simulink model "CarControl"  (R2022b)
settings: Solver=FixedStepDiscrete  StartTime=0.0  StopTime=10.0  FixedStep=0.01  RelTol=1e-3
libraries: simulink x9, simulink_extras x1
settings Model: Creator=Admin  LastModifiedBy=lu
settings OptimizationCC: DefaultParameterBehavior=Inlined  UseDivisionForNetSlopeComputation=on  GainParamInheritBuiltInType=on  UseFloatMulNetSlope=on  InlineInvariantSignals=on  PassReuseOutputArgsAs=Individual arguments  ZeroExternalMemoryAtStartup=off  ZeroInternalMemoryAtStartup=off  NoFixptDivByZeroProtection=on  EfficientFloat2IntCast=on  LifeSpan=1  OptimizeBlockOrder=speed  DifferentSizesBufferReuse=on  EfficientTunableParamExpr=on
settings DebuggingCC: ParameterTunabilityLossMsg=error  UnconnectedInputMsg=warning  UnconnectedOutputMsg=warning  UnconnectedLineMsg=warning
settings HardwareCC: ProdLongLongMode=on
settings SFSimCC: MATLABDynamicMemAlloc=off
settings RTWCC: Description=Embedded Coder  SystemTargetFile=ert.tlc  PackageName=RemoteControllerCodeGen  TemplateMakefile=ert_default_tmf  DLArmComputeVersion=19.05
settings CodeAppCC: ForceParamTrailComments=on  IgnoreCustomStorageClasses=off  OperatorAnnotations=on  SimulinkDataObjDesc=on  SFDataObjDesc=on  CustomSymbolStrGlobalVar=rt$N$M  CustomSymbolStrType=$N$M  CustomSymbolStrFcn=$N$M$F  CustomSymbolStrMacro=$N$M  InsertBlockDesc=on
settings ERTTargetCC: TargetLangStandard=C99 (ISO)  GenerateSampleERTMain=on  IncludeMdlTerminateFcn=off  CombineSignalStateStructs=on  SupportAbsoluteTime=off  SupportComplex=off  SupportNonInlinedSFcns=on  InlinedParameterPlacement=NonHierarchical  ERTCustomFileTemplate=example_file_process.tlc  ERTFilePackagingFormat=CompactWithDataFile

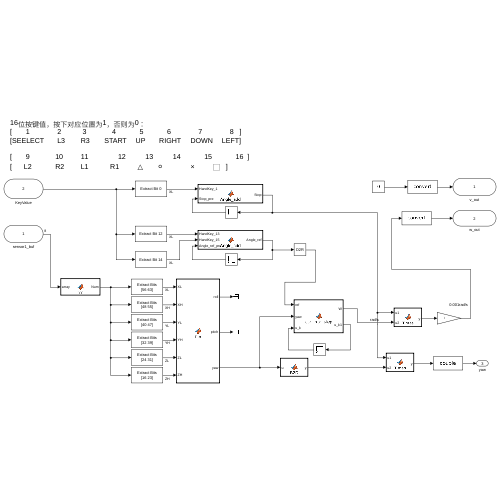
[thumbnail: Simulink's stored preview of the top-level diagram]
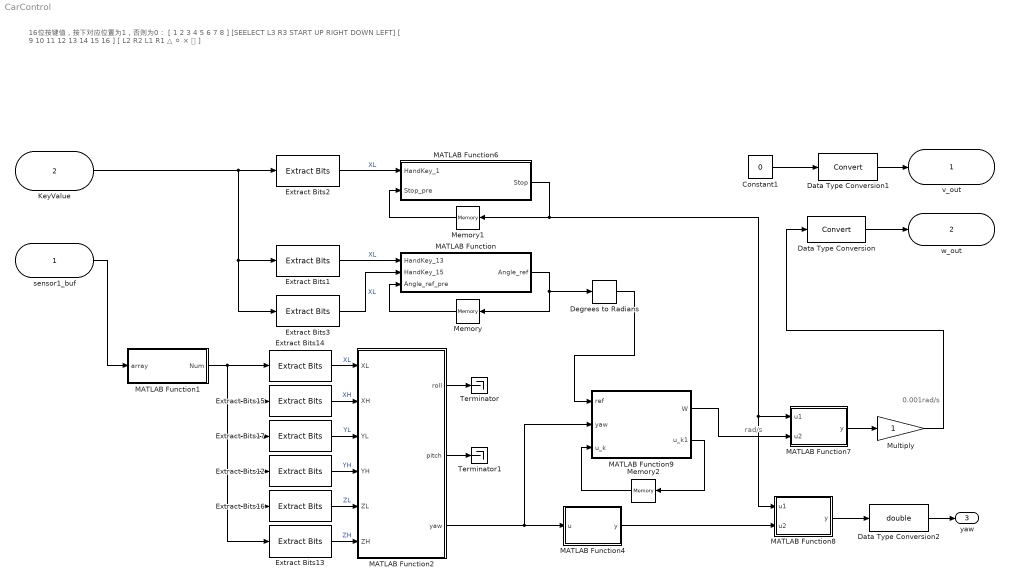
== system CarControl ==
  note: 16位按键值，按下对应位置为1，否则为0：
      | [ 1 2 3 4 5 6 7 8 ]
      | [SEELECT L3 R3 START UP RIGHT DOWN LEFT]
      |
      | [ 9 10 11 12 13 14 15 16 ]
      | [ L2 R2 L1 R1 △ ⚪ × ⃞ ]
  note: 0.001rad/s
  note: rad/s
  sensor1_buf : Inport  OutDataTypeStr=int8  PortDimensions=8
  KeyValue : Inport  Port=2  OutDataTypeStr=uint16  PortDimensions=1
  Constant1 : Constant  Value=0  OutDataTypeStr=uint8  SampleTime=-1
  Data Type Conversion : DataTypeConversion  SaturateOnIntegerOverflow=off  RndMeth=Floor
  Data Type Conversion1 : DataTypeConversion  SaturateOnIntegerOverflow=off  RndMeth=Floor
  Data Type Conversion2 : DataTypeConversion  OutDataTypeStr=double  SaturateOnIntegerOverflow=off  RndMeth=Floor
  Degrees to Radians : simulink_extras/Transformations/Degrees to Radians
  Extract Bits1 : simulink/Logic and Bit Operations/Extract Bits  bitsToExtract=Range of bits  numBits=8  bitIdxRange=[12]  outScalingMode=Treat bit field as an integer
  Extract Bits12 : simulink/Logic and Bit Operations/Extract Bits  bitsToExtract=Range of bits  numBits=8  bitIdxRange=[32 39]  outScalingMode=Treat bit field as an integer
  Extract Bits13 : simulink/Logic and Bit Operations/Extract Bits  bitsToExtract=Range of bits  numBits=8  bitIdxRange=[16 23]  outScalingMode=Treat bit field as an integer
  Extract Bits14 : simulink/Logic and Bit Operations/Extract Bits  bitsToExtract=Range of bits  numBits=8  bitIdxRange=[56 63]  outScalingMode=Treat bit field as an integer
  Extract Bits15 : simulink/Logic and Bit Operations/Extract Bits  bitsToExtract=Range of bits  numBits=8  bitIdxRange=[48 55]  outScalingMode=Treat bit field as an integer
  Extract Bits16 : simulink/Logic and Bit Operations/Extract Bits  bitsToExtract=Range of bits  numBits=8  bitIdxRange=[24 31]  outScalingMode=Treat bit field as an integer
  Extract Bits17 : simulink/Logic and Bit Operations/Extract Bits  bitsToExtract=Range of bits  numBits=8  bitIdxRange=[40 47]  outScalingMode=Treat bit field as an integer
  Extract Bits2 : simulink/Logic and Bit Operations/Extract Bits  bitsToExtract=Range of bits  numBits=8  bitIdxRange=[0]  outScalingMode=Treat bit field as an integer
  Extract Bits3 : simulink/Logic and Bit Operations/Extract Bits  bitsToExtract=Range of bits  numBits=8  bitIdxRange=[14]  outScalingMode=Treat bit field as an integer
  MATLAB Function : MATLAB Function  TreatAsAtomicUnit=on
  MATLAB Function1 : MATLAB Function  TreatAsAtomicUnit=on
  MATLAB Function2 : MATLAB Function  TreatAsAtomicUnit=on
  MATLAB Function4 : MATLAB Function  TreatAsAtomicUnit=on
  MATLAB Function6 : MATLAB Function  TreatAsAtomicUnit=on
  MATLAB Function7 : MATLAB Function  TreatAsAtomicUnit=on
  MATLAB Function8 : MATLAB Function  TreatAsAtomicUnit=on
  MATLAB Function9 : MATLAB Function  TreatAsAtomicUnit=on
  Memory : Memory
  Memory1 : Memory
  Memory2 : Memory
  Multiply : Gain  OutDataTypeStr=double
  Terminator : Terminator
  Terminator1 : Terminator
  v_out : Outport  OutDataTypeStr=double
  w_out : Outport  Port=2  OutDataTypeStr=double
  yaw : Outport  Port=3  OutDataTypeStr=double
  wires:
  Extract Bits14/1 -> MATLAB Function2/1(XL)  "XL"
  Extract Bits15/1 -> MATLAB Function2/2(XH)  "XH"
  Extract Bits17/1 -> MATLAB Function2/3(YL)  "YL"
  Extract Bits13/1 -> MATLAB Function2/6(ZH)  "ZH"
  Extract Bits12/1 -> MATLAB Function2/4(YH)  "YH"
  Extract Bits16/1 -> MATLAB Function2/5(ZL)  "ZL"
  MATLAB Function1/1(Num) -> Extract Bits13/1, Extract Bits16/1, Extract Bits12/1, Extract Bits17/1, Extract Bits15/1, Extract Bits14/1
  Constant1/1 -> Data Type Conversion1/1
  Multiply/1 -> Data Type Conversion/1
  Data Type Conversion/1 -> w_out/1
  Data Type Conversion1/1 -> v_out/1
  Data Type Conversion2/1 -> yaw/1
  MATLAB Function2/2(pitch) -> Terminator1/1
  MATLAB Function2/1(roll) -> Terminator/1
  MATLAB Function2/3(yaw) -> MATLAB Function9/2(yaw), MATLAB Function4/1(u)
  sensor1_buf/1 -> MATLAB Function1/1(array)
  KeyValue/1 -> Extract Bits3/1, Extract Bits1/1, Extract Bits2/1
  Extract Bits1/1 -> MATLAB Function/1(HandKey_13)  "XL"
  MATLAB Function/1(Angle_ref) -> Memory/1, Degrees to Radians/1
  Memory/1 -> MATLAB Function/3(Angle_ref_pre)
  Extract Bits2/1 -> MATLAB Function6/1(HandKey_1)  "XL"
  Memory1/1 -> MATLAB Function6/2(Stop_pre)
  MATLAB Function9/1(W) -> MATLAB Function7/2(u2)
  MATLAB Function7/1(y) -> Multiply/1
  MATLAB Function4/1(y) -> MATLAB Function8/2(u2)
  MATLAB Function8/1(y) -> Data Type Conversion2/1
  MATLAB Function6/1(Stop) -> MATLAB Function8/1(u1), MATLAB Function7/1(u1), Memory1/1
  Degrees to Radians/1 -> MATLAB Function9/1(ref)
  Extract Bits3/1 -> MATLAB Function/2(HandKey_15)  "XL"
  MATLAB Function9/2(u_k1) -> Memory2/1
  Memory2/1 -> MATLAB Function9/3(u_k)

== matlab function CarControl/MATLAB Function1 ==
  data: array input; Num output
function Num = fcn(array)
Num=int64(0);
len = length(array);
    for i=1:len
            Num = bitshift(Num,8)+int64(array(i));
    end
Num = int64(Num);
end

== matlab function CarControl/MATLAB Function ==
  data: HandKey_13 input; HandKey_15 input; Angle_ref output; Angle_ref_pre input
function Angle_ref = Angle_add(HandKey_13,HandKey_15,Angle_ref_pre)

Angle_ref = 0;

if HandKey_13 == 0
    Angle_ref = Angle_ref_pre + 3;
    if Angle_ref >= 350
        Angle_ref = 350;
    end
elseif HandKey_15 == 0
    Angle_ref = Angle_ref_pre - 3;
    if Angle_ref <= 10
        Angle_ref = 10;
    end
else
    Angle_ref = Angle_ref_pre;
end

== matlab function CarControl/MATLAB Function4 ==
  data: u input; y output
function y = R2D(u)

y = double(u)/pi*180;

== matlab function CarControl/MATLAB Function6 ==
  data: HandKey_1 input; Stop output; Stop_pre input
function Stop = Angle_add(HandKey_1,Stop_pre)

Stop = 0;
Stop = Stop_pre;
if HandKey_1 == 0
    if Stop_pre == 0
        Stop = 1;
    else
        Stop = 0;
    end
end

== matlab function CarControl/MATLAB Function7 ==
  data: u1 input; y output; u2 input
function y = Times(u1,u2)

y = u1*u2;

== matlab function CarControl/MATLAB Function8 ==
  data: u1 input; y output; u2 input
function y = Times(u1,u2)

y = u1*u2;

== matlab function CarControl/MATLAB Function9 ==
  data: ref input; W output; yaw input; u_k input; u_k1 output
function [W,u_k1] = car_mpc_step(ref, yaw, u_k)

    % 更新系统模型
    A = [0, 0, -u_k(1, 1) * sin(yaw); ...
             0, 0, u_k(1, 1) * cos(yaw); ...
             0, 0, 0];
    B = [cos(yaw), 0; ...
             sin(yaw), 0; ...
             0, 1];

    % 定义权重矩阵
    Q = eye(3);
    Q(1, 1) = 1000;
    Q(2, 2) = 1000;
    Q(3, 3) = 100;
    R = eye(2);
    R(1, 1) = 1;
    R(2, 2) = 1;
    F = Q;

    C = eye(3);
    D = zeros(3, 2);
    % 系统离散化
    Ts = 0.002;
    sys_c = ss(A, B, C, D);
    sys_d = c2d(sys_c, Ts);

    % 定义控制区间
    n_steps = 5;

    % 定义状态矩阵 A, n x n 矩阵
    n = size(sys_d.A, 1); %取其行数，即状态空间变量个数

    % 定义输入矩阵 B, n x p 矩阵
    p = size(sys_d.B, 2); %取其列数，即输入变量个数

    % 当前状态变量值， n x 1 向量
    X_K = [0; 0; yaw];

    % 获得期望目标
    y_t = [0; 0; ref];

    %定义目标向量
    Y_T = y_t;

    for i = 0:n_steps

        for j = 1:n
            Y_K((i * n + j), 1) = Y_T(j, 1);
        end

    end

    % Call MPC_Matrices 函数 求得 E,H矩阵
    [E, L, H] = MPC_Matrices(sys_d.A, sys_d.B, Q, R, F, n_steps);

    % 求解二次规划问题得输出
    u_k1 = Prediction(Y_K, X_K, E, L, H, n_steps, p);
    W = u_k1(2,1);

== matlab function CarControl/MATLAB Function2 ==
  data: roll output; pitch output; yaw output; XL input; XH input; YL input; YH input; ZL input; ZH input
function [roll,pitch,yaw] = fcn(XL,XH,YL,YH,ZL,ZH)
XL = int16(XL);
XH = int16(XH);
YL = int16(YL);
YH = int16(YH);
ZL = int16(ZL);
ZH = int16(ZH);
a=bitshift(XH,8)+XL;
b=bitshift(YH,8)+YL;
c=int16(bitshift(ZH,8))+int16(ZL);
roll=double(a)*pi/(100*180);
pitch=double(b)*pi/(100*180);
yaw=double(c)*pi/(100*180);
